simulink model "pruebas_of_modelo_completo"  (R2021a)
settings: Solver=VariableStepAuto  StartTime=0.0  StopTime=10.0  RelTol=1e-3
undefined symbols (not defined in the file): bah, bat, bcx, bcy, beqh, beqhd, beqt, bw, cont_mass, ddxmax, ddxmin, g, Kcy, Ksah, Ksat, Ksiah, Ksiat, Kw, Meqh, Meqt, Rd, rt, rth, Rw, sp_mass, yt0
settings Model: Creator=Mariano  LastModifiedBy=facu_

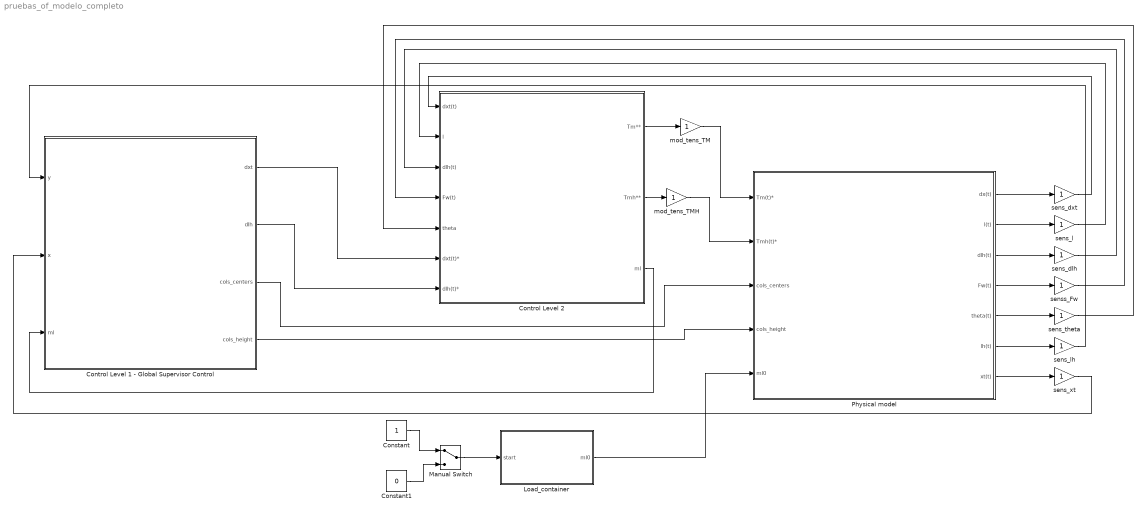
== system pruebas_of_modelo_completo ==
  Constant : Constant
  Constant1 : Constant  Value=0
  Control Level 1 - Global Supervisor Control : Stateflow chart  TreatAsAtomicUnit=on
  Control Level 2 : Subsystem
  Load_container : Subsystem
  Manual Switch : ManualSwitch
  Physical model : Subsystem
  mod_tens_TM : Gain
  mod_tens_TMH : Gain
  sens_dlh : Gain
  sens_dxt : Gain
  sens_l : Gain
  sens_lh : Gain
  sens_theta : Gain
  sens_xt : Gain
  senss_Fw : Gain
  wires:
  Control Level 2/1(Tm**) -> mod_tens_TM/1
  Control Level 2/2(Tmh**) -> mod_tens_TMH/1
  Control Level 1 - Global Supervisor Control/1(dxt) -> Control Level 2/6(dxt(t)*)
  Control Level 1 - Global Supervisor Control/2(dlh) -> Control Level 2/7(dlh(t)*)
  Physical model/1(dx(t)) -> sens_dxt/1
  Physical model/2(l(t)) -> sens_l/1
  Physical model/3(dlh(t)) -> sens_dlh/1
  Physical model/4(Fw(t)) -> senss_Fw/1
  Physical model/5(theta(t)) -> sens_theta/1
  Physical model/6(lh(t)) -> sens_lh/1
  Physical model/7(xt(t)) -> sens_xt/1
  sens_dxt/1 -> Control Level 2/1(dxt(t))
  sens_l/1 -> Control Level 2/2(l)
  sens_dlh/1 -> Control Level 2/3(dlh(t))
  senss_Fw/1 -> Control Level 2/4(Fw(t))
  sens_theta/1 -> Control Level 2/5(theta)
  sens_lh/1 -> Control Level 1 - Global Supervisor Control/1(y)
  sens_xt/1 -> Control Level 1 - Global Supervisor Control/2(x)
  mod_tens_TM/1 -> Physical model/1(Tm(t)*)
  mod_tens_TMH/1 -> Physical model/2(Tmh(t)*)
  Control Level 1 - Global Supervisor Control/3(cols_centers) -> Physical model/3(cols_centers)
  Control Level 1 - Global Supervisor Control/4(cols_height) -> Physical model/4(cols_height)
  Load_container/1(ml0) -> Physical model/5(ml0)
  Manual Switch/1 -> Load_container/1(start)
  Constant/1 -> Manual Switch/1
  Constant1/1 -> Manual Switch/2
  Control Level 2/3(ml) -> Control Level 1 - Global Supervisor Control/3(ml)

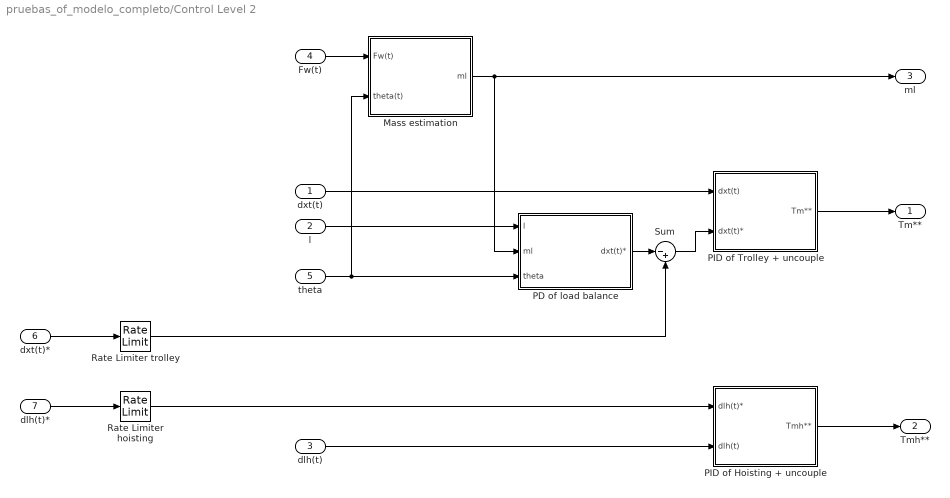
== system pruebas_of_modelo_completo/Control Level 2 ==
  dxt(t) : Inport
  l : Inport  Port=2
  dlh(t) : Inport  Port=3
  Fw(t) : Inport  Port=4
  theta : Inport  Port=5
  dxt(t)* : Inport  Port=6
  dlh(t)* : Inport  Port=7
  Mass estimation : Subsystem
  "PD of load balance " : Subsystem
  "PID of Hoisting + uncouple " : Subsystem
  "PID of Trolley + uncouple " : Subsystem
  Rate Limiter hoisting : RateLimiter  RisingSlewLimit=ddxmax  FallingSlewLimit=ddxmin
  Rate Limiter trolley : RateLimiter  RisingSlewLimit=ddxmax  FallingSlewLimit=ddxmin
  Sum : Sum  Inputs=|-+
  Tm** : Outport
  Tmh** : Outport  Port=2
  ml : Outport  Port=3
  wires:
  dlh(t)*/1 -> Rate Limiter hoisting/1
  Fw(t)/1 -> Mass estimation/1(Fw(t))
  "PID of Trolley + uncouple "/1(Tm**) -> Tm**/1
  Mass estimation/1(ml) -> ml/1, "PD of load balance "/2(ml)
  "PD of load balance "/1(dxt(t)*) -> Sum/1
  Sum/1 -> "PID of Trolley + uncouple "/2(dxt(t)*)
  dxt(t)/1 -> "PID of Trolley + uncouple "/1(dxt(t))
  "PID of Hoisting + uncouple "/1(Tmh**) -> Tmh**/1
  dxt(t)*/1 -> Rate Limiter trolley/1
  l/1 -> "PD of load balance "/1(l)
  theta/1 -> Mass estimation/2(theta(t)), "PD of load balance "/3(theta)
  Rate Limiter trolley/1 -> Sum/2
  Rate Limiter hoisting/1 -> "PID of Hoisting + uncouple "/1(dlh(t)*)
  dlh(t)/1 -> "PID of Hoisting + uncouple "/2(dlh(t))

== system pruebas_of_modelo_completo/Load_container ==
  start : Inport
  Sum : Sum  Inputs=|++
  Switch : Switch  Criteria=u2 > Threshold
  no_container : Constant  Value=0
  random_container_mass : Constant  Value=cont_mass
  spreader mass : Constant  Value=sp_mass
  ml0 : Outport
  wires:
  no_container/1 -> Switch/1
  spreader mass/1 -> Sum/2
  random_container_mass/1 -> Switch/3
  Switch/1 -> Sum/1
  Sum/1 -> ml0/1
  start/1 -> Switch/2

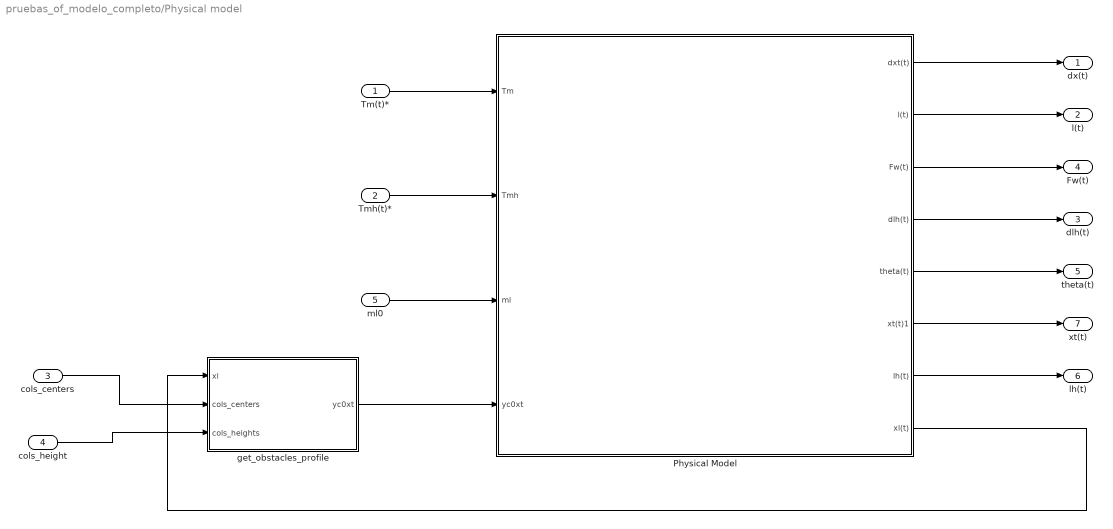
== system pruebas_of_modelo_completo/Physical model ==
  Tm(t)* : Inport
  Tmh(t)* : Inport  Port=2
  cols_centers : Inport  Port=3
  cols_height : Inport  Port=4
  ml0 : Inport  Port=5
  Physical Model : Subsystem
  get_obstacles_profile : MATLAB Function  TreatAsAtomicUnit=on
  dx(t) : Outport
  l(t) : Outport  Port=2
  dlh(t) : Outport  Port=3
  Fw(t) : Outport  Port=4
  theta(t) : Outport  Port=5
  lh(t) : Outport  Port=6
  xt(t) : Outport  Port=7
  wires:
  Physical Model/4(dlh(t)) -> dlh(t)/1
  Physical Model/2(l(t)) -> l(t)/1
  Physical Model/1(dxt(t)) -> dx(t)/1
  Physical Model/3(Fw(t)) -> Fw(t)/1
  Physical Model/5(theta(t)) -> theta(t)/1
  Physical Model/6(xt(t)1) -> xt(t)/1
  Physical Model/7(lh(t)) -> lh(t)/1
  Tmh(t)*/1 -> Physical Model/2(Tmh)
  Tm(t)*/1 -> Physical Model/1(Tm)
  ml0/1 -> Physical Model/3(ml)
  get_obstacles_profile/1(yc0xt) -> Physical Model/4(yc0xt)
  Physical Model/8(xl(t)) -> get_obstacles_profile/1(xl)
  cols_centers/1 -> get_obstacles_profile/2(cols_centers)
  cols_height/1 -> get_obstacles_profile/3(cols_heights)

== system pruebas_of_modelo_completo/Control Level 2/Mass estimation ==
  Fw(t) : Inport
  theta(t) : Inport  Port=2
  Constant : Constant  Value=g
  Divide : Product  Inputs=*/
  Product : Product
  Trigonometric Function : Trigonometry
  ml : Outport
  wires:
  theta(t)/1 -> Trigonometric Function/1
  Trigonometric Function/1 -> Product/2
  Fw(t)/1 -> Product/1
  Divide/1 -> ml/1
  Product/1 -> Divide/1
  Constant/1 -> Divide/2

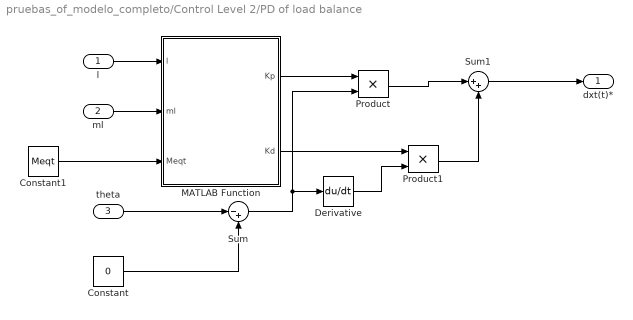
== system pruebas_of_modelo_completo/Control Level 2/PD of load balance  ==
  l : Inport
  ml : Inport  Port=2
  theta : Inport  Port=3
  Constant : Constant  Value=0
  Constant1 : Constant  Value=Meqt
  Derivative : Derivative
  MATLAB Function : MATLAB Function  TreatAsAtomicUnit=on
  Product : Product
  Product1 : Product
  Sum : Sum  Inputs=|-+
  Sum1 : Sum  Inputs=|++
  dxt(t)* : Outport
  wires:
  theta/1 -> Sum/1
  Constant/1 -> Sum/2
  ml/1 -> MATLAB Function/2(ml)
  Sum/1 -> Product/2, Derivative/1
  Product1/1 -> Sum1/2
  Product/1 -> Sum1/1
  Sum1/1 -> dxt(t)*/1
  MATLAB Function/2(Kd) -> Product1/1
  MATLAB Function/1(Kp) -> Product/1
  Derivative/1 -> Product1/2
  l/1 -> MATLAB Function/1(l)
  Constant1/1 -> MATLAB Function/3(Meqt)

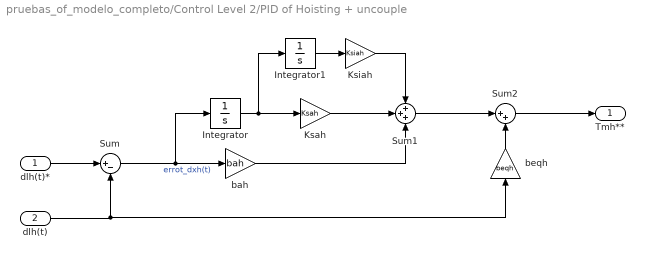
== system pruebas_of_modelo_completo/Control Level 2/PID of Hoisting + uncouple  ==
  dlh(t)* : Inport
  dlh(t) : Inport  Port=2
  Integrator : Integrator
  Integrator1 : Integrator
  Ksah : Gain  Gain=Ksah
  Ksiah : Gain  Gain=Ksiah
  Sum : Sum  Inputs=|+-
  Sum1 : Sum  Inputs=+++
  Sum2 : Sum  Inputs=|++
  bah : Gain  Gain=bah
  beqh : Gain  Gain=beqh
  Tmh** : Outport
  wires:
  Sum/1 -> bah/1, Integrator/1  "errot_dxh(t)"
  dlh(t)*/1 -> Sum/1
  Sum1/1 -> Sum2/1
  dlh(t)/1 -> beqh/1, Sum/2
  Integrator/1 -> Integrator1/1, Ksah/1
  bah/1 -> Sum1/3
  Ksah/1 -> Sum1/2
  Integrator1/1 -> Ksiah/1
  Ksiah/1 -> Sum1/1
  beqh/1 -> Sum2/2
  Sum2/1 -> Tmh**/1

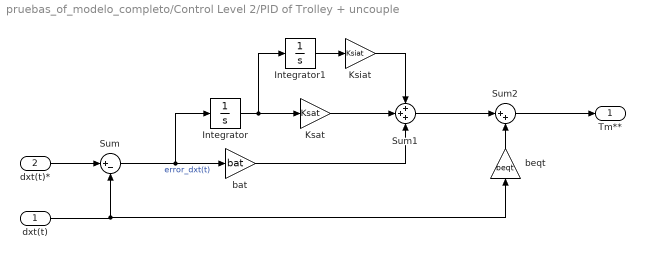
== system pruebas_of_modelo_completo/Control Level 2/PID of Trolley + uncouple  ==
  dxt(t) : Inport
  dxt(t)* : Inport  Port=2
  Integrator : Integrator
  Integrator1 : Integrator
  Ksat : Gain  Gain=Ksat
  Ksiat : Gain  Gain=Ksiat
  Sum : Sum  Inputs=|+-
  Sum1 : Sum  Inputs=+++
  Sum2 : Sum  Inputs=|++
  bat : Gain  Gain=bat
  beqt : Gain  Gain=beqt
  Tm** : Outport
  wires:
  Sum/1 -> bat/1, Integrator/1  "error_dxt(t)"
  dxt(t)*/1 -> Sum/1
  Sum1/1 -> Sum2/1
  dxt(t)/1 -> beqt/1, Sum/2
  Integrator/1 -> Integrator1/1, Ksat/1
  bat/1 -> Sum1/3
  Ksat/1 -> Sum1/2
  Integrator1/1 -> Ksiat/1
  Ksiat/1 -> Sum1/1
  beqt/1 -> Sum2/2
  Sum2/1 -> Tm**/1

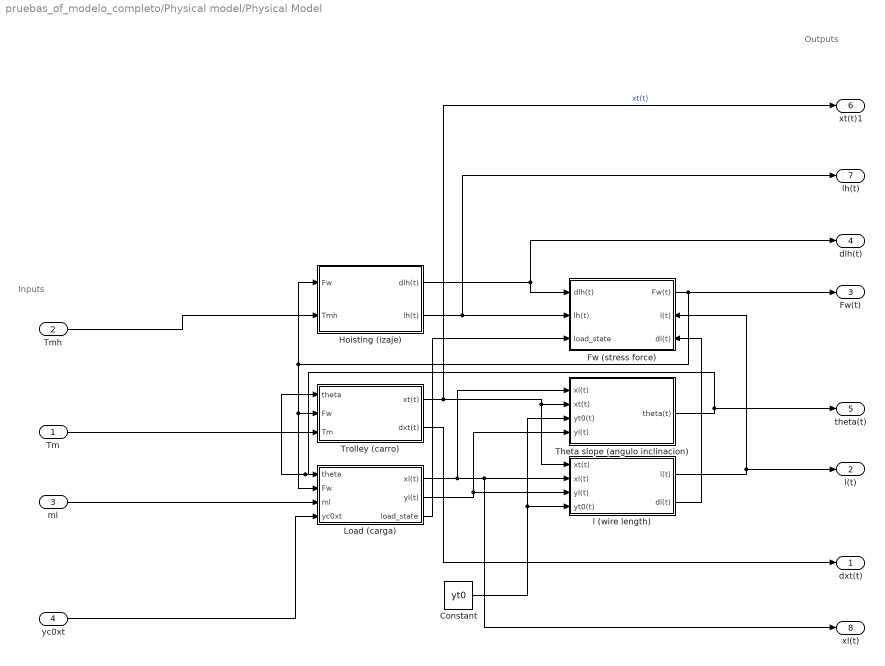
== system pruebas_of_modelo_completo/Physical model/Physical Model ==
  note: Inputs
  note: Outputs
  Tm : Inport
  Tmh : Inport  Port=2
  ml : Inport  Port=3
  yc0xt : Inport  Port=4
  Constant : Constant  Value=yt0
  Fw (stress force) : Subsystem
      settings: PortSchema="{\"entries\":[{\"content\":{\"sides\":[{\"content\":{\"connectorIds\":[\"In1\",\"In2\",\"In3\"]},\"type\":\"ConnectorPlacement.EquallySpacedRectSide\",\"uuid\":\"ba23d8a5-df88-4a98-9228-1a95ef0572d6\"},{\"content\":{\"connectorIds\":[\"Out1\",\"In4\",\"In5\"],\"side\":\"RIGHT\"},\"type\":\"ConnectorPlacement.EquallySpacedRectSide\",\"uuid\":\"c1b2cc2a-1d19-40da-89ec-405abbf25b58\"},{\"content\":{\"connectorIds\":[],\"side\":\"TOP\"},\"type\":\"ConnectorPlacement.EquallySpacedRectSide\",\"uuid\":\"8c283652-7118-429a-8320-3bc0966db205\"}]},\"type\":\"ConnectorPlacement.EquallySpacedConnector\",\"uuid\":\"7ebc4a5f-6f80-4333-9ee6-9a21b2f2a5d0\"}],\"packageUris\":[\"http://schema.mathworks.com/mf0/Connector/R2020b\"],\"version\":\"1.0\"}"
  Hoisting (izaje) : Subsystem
  Load (carga) : Subsystem
  Theta slope (angulo inclinacion) : Subsystem
  Trolley (carro) : Subsystem
  l (wire length) : Subsystem
  dxt(t) : Outport
  l(t) : Outport  Port=2
  Fw(t) : Outport  Port=3
  dlh(t) : Outport  Port=4
  theta(t) : Outport  Port=5
  xt(t)1 : Outport  Port=6
  lh(t) : Outport  Port=7
  xl(t) : Outport  Port=8
  wires:
  Theta slope (angulo inclinacion)/1(theta(t)) -> theta(t)/1, Trolley (carro)/1(theta), Load (carga)/1(theta)
  Load (carga)/1(xl(t)) -> xl(t)/1, l (wire length)/2(xl(t)), Theta slope (angulo inclinacion)/1(xl(t))
  Hoisting (izaje)/2(lh(t)) -> lh(t)/1, Fw (stress force)/2(lh(t))
  Trolley (carro)/1(xt(t)) -> xt(t)1/1, l (wire length)/1(xt(t)), Theta slope (angulo inclinacion)/2(xt(t))  "xt(t)"
  Fw (stress force)/1(Fw(t)) -> Trolley (carro)/2(Fw), Load (carga)/2(Fw), Hoisting (izaje)/1(Fw), Fw(t)/1
  Constant/1 -> Theta slope (angulo inclinacion)/3(yt0(t)), l (wire length)/4(yt0(t))
  Load (carga)/2(yl(t)) -> Theta slope (angulo inclinacion)/4(yl(t)), l (wire length)/3(yl(t))
  l (wire length)/1(l(t)) -> l(t)/1, Fw (stress force)/4(l(t))
  ml/1 -> Load (carga)/3(ml)
  l (wire length)/2(dl(t)) -> Fw (stress force)/5(dl(t))
  Tmh/1 -> Hoisting (izaje)/2(Tmh)
  Tm/1 -> Trolley (carro)/3(Tm)
  Hoisting (izaje)/1(dlh(t)) -> Fw (stress force)/1(dlh(t)), dlh(t)/1
  Trolley (carro)/2(dxt(t)) -> dxt(t)/1
  Load (carga)/3(load_state) -> Fw (stress force)/3(load_state)
  yc0xt/1 -> Load (carga)/4(yc0xt)

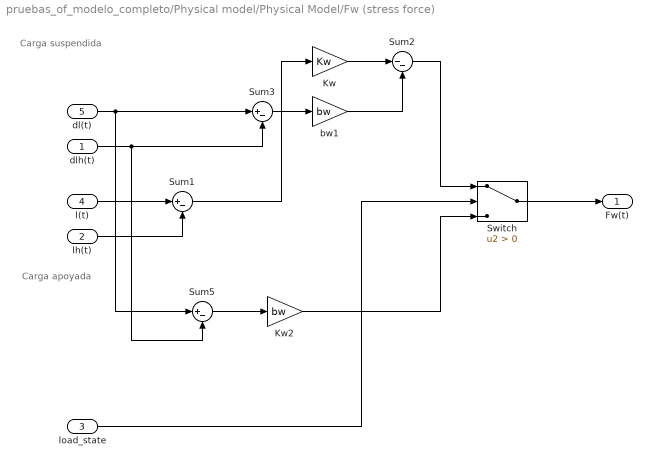
== system pruebas_of_modelo_completo/Physical model/Physical Model/Fw (stress force) ==
  note: Carga suspendida
  note: Carga apoyada
  dlh(t) : Inport
  lh(t) : Inport  Port=2
  load_state : Inport  Port=3
  l(t) : Inport  Port=4
  dl(t) : Inport  Port=5
  Kw : Gain  Gain=Kw
  Kw2 : Gain  Gain=bw
  Sum1 : Sum  Inputs=|+-
  Sum2 : Sum  Inputs=|--
  Sum3 : Sum  Inputs=|+-
  Sum5 : Sum  Inputs=|+-
  Switch : Switch  Criteria=u2 > Threshold
  bw1 : Gain  Gain=bw
  Fw(t) : Outport
  wires:
  Switch/1 -> Fw(t)/1
  l(t)/1 -> Sum1/1
  lh(t)/1 -> Sum1/2
  Sum1/1 -> Kw/1
  Sum3/1 -> bw1/1
  bw1/1 -> Sum2/2
  Kw/1 -> Sum2/1
  Sum2/1 -> Switch/1
  Sum5/1 -> Kw2/1
  dlh(t)/1 -> Sum5/2, Sum3/2
  dl(t)/1 -> Sum5/1, Sum3/1
  Kw2/1 -> Switch/3
  load_state/1 -> Switch/2

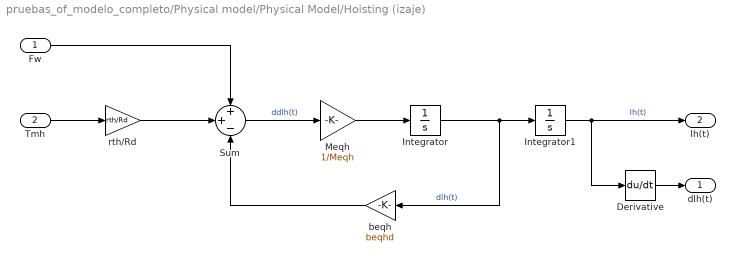
== system pruebas_of_modelo_completo/Physical model/Physical Model/Hoisting (izaje) ==
  Fw : Inport
  Tmh : Inport  Port=2
  Derivative : Derivative
  Integrator : Integrator
  Integrator1 : Integrator
  Meqh : Gain  Gain=1/Meqh
  Sum : Sum  Inputs=++-
  beqh : Gain  Gain=beqhd
  rth/Rd : Gain  Gain=rth/Rd
  dlh(t) : Outport
  lh(t) : Outport  Port=2
  wires:
  Fw/1 -> Sum/1
  Tmh/1 -> rth/Rd/1
  rth/Rd/1 -> Sum/2
  Sum/1 -> Meqh/1  "ddlh(t)"
  Meqh/1 -> Integrator/1
  Integrator/1 -> beqh/1, Integrator1/1  "dlh(t)"
  Integrator1/1 -> Derivative/1, lh(t)/1  "lh(t)"
  beqh/1 -> Sum/3
  Derivative/1 -> dlh(t)/1

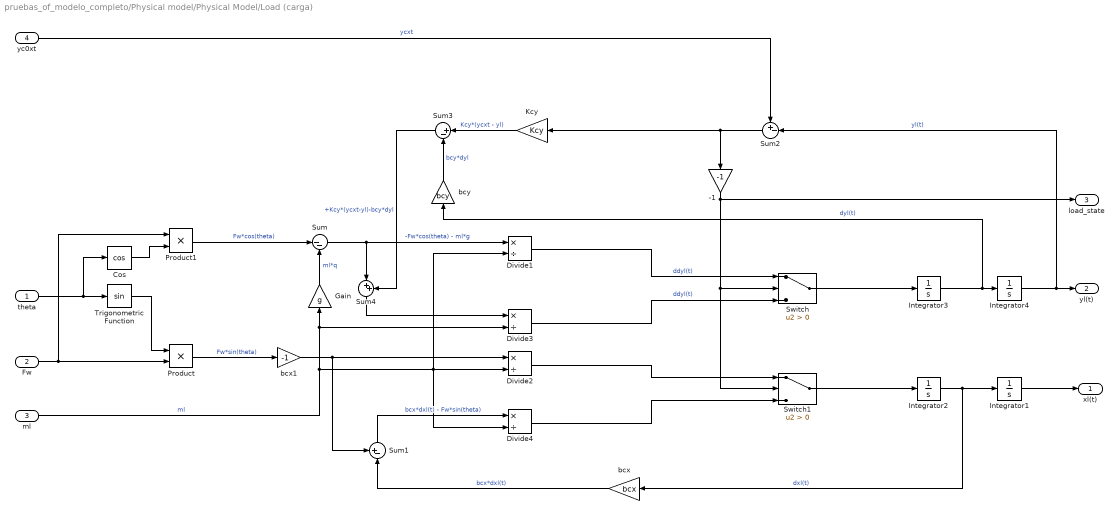
== system pruebas_of_modelo_completo/Physical model/Physical Model/Load (carga) ==
  theta : Inport
  Fw : Inport  Port=2
  ml : Inport  Port=3
  yc0xt : Inport  Port=4
  -1 : Gain  Gain=-1
  Cos : Trigonometry  Operator=cos
  Divide{1..4} (4 alike) : Product  Inputs=*/
  Gain : Gain  Gain=g
  Integrator{1..4} (4 alike) : Integrator
  Kcy : Gain  Gain=Kcy
  Product : Product
  Product1 : Product
  Sum : Sum  Inputs=|--
  Sum1 : Sum  Inputs=+-|
  Sum2 : Sum  Inputs=+-|
  Sum3 : Sum  Inputs=|+-
  Sum4 : Sum  Inputs=|++
  Switch : Switch  Criteria=u2 > Threshold
  Switch1 : Switch  Criteria=u2 > Threshold
  Trigonometric Function : Trigonometry
  bcx : Gain  Gain=bcx
  bcx1 : Gain  Gain=-1
  bcy : Gain  Gain=bcy
  xl(t) : Outport
  yl(t) : Outport  Port=2
  load_state : Outport  Port=3
  wires:
  theta/1 -> Trigonometric Function/1, Cos/1
  Trigonometric Function/1 -> Product/1
  Fw/1 -> Product/2, Product1/1
  Integrator1/1 -> xl(t)/1
  Integrator2/1 -> bcx/1, Integrator1/1  "dxl(t)"
  ml/1 -> Divide4/2, Divide2/2, Divide1/2, Divide3/2, Gain/1  "ml"
  Product/1 -> bcx1/1  "Fw*sin(theta)"
  Cos/1 -> Product1/2
  Product1/1 -> Sum/1  "Fw*cos(theta)"
  Sum/1 -> Sum4/1, Divide1/1  "-Fw*cos(theta) - ml*g"
  Integrator3/1 -> bcy/1, Integrator4/1  "dyl(t)"
  Integrator4/1 -> Sum2/2, yl(t)/1  "yl(t)"
  Gain/1 -> Sum/2  "ml*q"
  Divide1/1 -> Switch/1  "ddyl(t)"
  Switch/1 -> Integrator3/1
  Switch1/1 -> Integrator2/1
  Divide2/1 -> Switch1/1
  Divide4/1 -> Switch1/3
  Divide3/1 -> Switch/3  "ddyl(t)"
  bcx1/1 -> Sum1/1, Divide2/1
  bcx/1 -> Sum1/2  "bcx*dxl(t)"
  Sum1/1 -> Divide4/1  "bcx*dxl(t) - Fw*sin(theta)"
  Sum2/1 -> Kcy/1, -1/1
  yc0xt/1 -> Sum2/1  "ycxt"
  Kcy/1 -> Sum3/1  "Kcy*(ycxt - yl)"
  bcy/1 -> Sum3/2  "bcy*dyl"
  Sum4/1 -> Divide3/1
  Sum3/1 -> Sum4/2  "+Kcy*(ycxt-yl)-bcy*dyl"
  -1/1 -> load_state/1, Switch1/2, Switch/2

== system pruebas_of_modelo_completo/Physical model/Physical Model/Theta slope (angulo inclinacion) ==
  xl(t) : Inport
  xt(t) : Inport  Port=2
  yt0(t) : Inport  Port=3
  yl(t) : Inport  Port=4
  Atan2 : Trigonometry  Operator=atan2
  Sum : Sum  Inputs=-+
  Sum1 : Sum  Inputs=+-
  theta(t) : Outport
  wires:
  yt0(t)/1 -> Sum/1
  yl(t)/1 -> Sum/2
  xl(t)/1 -> Sum1/1
  xt(t)/1 -> Sum1/2
  Sum1/1 -> Atan2/1  "xl-xt"
  Sum/1 -> Atan2/2  "yl-yt"
  Atan2/1 -> theta(t)/1

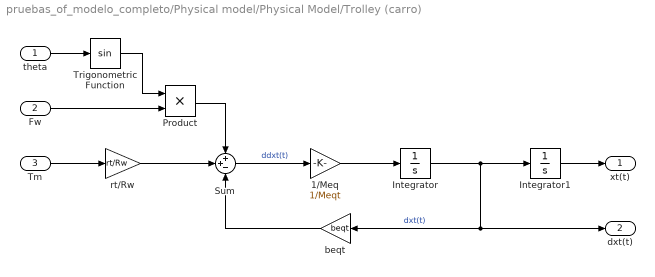
== system pruebas_of_modelo_completo/Physical model/Physical Model/Trolley (carro) ==
  theta : Inport
  Fw : Inport  Port=2
  Tm : Inport  Port=3
  1/Meq : Gain  Gain=1/Meqt
  Integrator : Integrator
  Integrator1 : Integrator
  Product : Product
  Sum : Sum  Inputs=++-
  Trigonometric Function : Trigonometry
  beqt : Gain  Gain=beqt
  rt/Rw : Gain  Gain=rt/Rw
  xt(t) : Outport
  dxt(t) : Outport  Port=2
  wires:
  theta/1 -> Trigonometric Function/1
  Trigonometric Function/1 -> Product/1
  Fw/1 -> Product/2
  Product/1 -> Sum/1
  Tm/1 -> rt/Rw/1
  rt/Rw/1 -> Sum/2
  Sum/1 -> 1/Meq/1  "ddxt(t)"
  1/Meq/1 -> Integrator/1
  Integrator/1 -> Integrator1/1, dxt(t)/1, beqt/1  "dxt(t)"
  Integrator1/1 -> xt(t)/1
  beqt/1 -> Sum/3

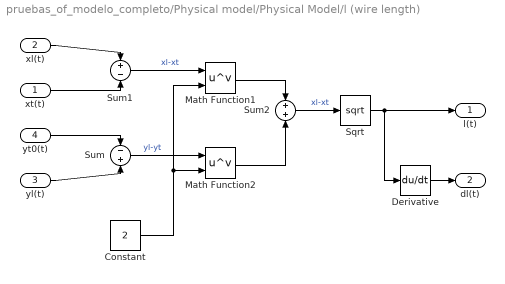
== system pruebas_of_modelo_completo/Physical model/Physical Model/l (wire length) ==
  xt(t) : Inport
  xl(t) : Inport  Port=2
  yl(t) : Inport  Port=3
  yt0(t) : Inport  Port=4
  Constant : Constant  Value=2
  Derivative : Derivative
  Math Function1 : Math  Operator=pow  SignedPower=on  SaturateOnIntegerOverflow=on
  Math Function2 : Math  Operator=pow  SignedPower=on  SaturateOnIntegerOverflow=on
  Sqrt : Sqrt  SaturateOnIntegerOverflow=on
  Sum : Sum  Inputs=-+
  Sum1 : Sum  Inputs=+-
  Sum2 : Sum
  l(t) : Outport
  dl(t) : Outport  Port=2
  wires:
  yt0(t)/1 -> Sum/1
  yl(t)/1 -> Sum/2
  xl(t)/1 -> Sum1/1
  xt(t)/1 -> Sum1/2
  Sqrt/1 -> Derivative/1, l(t)/1
  Sum1/1 -> Math Function1/1  "xl-xt"
  Sum/1 -> Math Function2/1  "yl-yt"
  Math Function1/1 -> Sum2/1
  Math Function2/1 -> Sum2/2
  Sum2/1 -> Sqrt/1  "xl-xt"
  Derivative/1 -> dl(t)/1
  Constant/1 -> Math Function2/2, Math Function1/2

== matlab function pruebas_of_modelo_completo/Control Level 2/PD of load balance /MATLAB Function ==
  data: l input; Kp output; ml input; Kd output; Meqt input
function [Kp,Kd] = fcn(l, ml,Meqt)
    wn=800;
    g=9.81;
    Kd = l - ( (Meqt*g)/((wn^2)*(ml+Meqt)) ) ;
    Kp = 2*wn*1*(-l + Kd);
end

== stateflow chart pruebas_of_modelo_completo/Control Level 1 - Global Supervisor Control ==
  note: Descripcion variables:
      | CARRO (TROLLEY):
      | - move_t -> (variable,int) boton para mover el carro en x.
      | - dx -> (variable,double) velocidad actual del carro (variable)
      | - VXt -> velocidad máxima del carro (es una constante, que al multiplicarla por bot_t modifica el valor de la velocidad real de carro.)
      | - limits_t -> (variable,bool) la variable cambia al valor 1 si se alcanzan los limites de movimiento del carro.
      |
      | IZAJE (HOISTING):
      | - move_h ->(variable,int) boton para izar la carga.
      | - dy -> (variable,double) velocidad actual del izaje.
      | - VYh -> (constante) velocidad máxima que puede alcanzar el izaje.
      | - limits_h -> (variable,bool) la variable cambia al valor 1 si se alcanzan los limites de movimiento del izaje.
      |
      | Descripcion de bloques:
      | - ALL_MANUAL:
      | Es el modo manual por defecto, el operario puede manejar el trolley y el hoisting con 2 botones. El boton move_t se encarga de mover el trolley y el boton move_h de izar la carga.
      | - HYRBID_MANUAL:
      | Es el modo manual que esta presente en los ciclos simple o doble. Es decir, esta intercalado con el modo automático
  note: Descripción de ciclos:
      | -SIMPLE:
      | O se carga o se descarga, es decir: Si estoy cargando el barco, en el tramo muelle -> barco llevo un contenedor, pero vuelvo vacio. Es decir que el tramo barco -> muelle es sin ningun contenedor. Lo mismo sucederia si estoy descargando el barco: el tramo barco -> muelle es con un contenedor cargado, pero el tramo muelle -> barco es en vacio.
      | - DOBLE:
      | Se puede cargar y descargar en el mismo ciclo de trabajo. Es decir, que el tramo muelle -> barco es con un contenedor cargado, y el tramo barco -> muelle también. Por ende, se permite una carga intermedia antes de volver al muelle.
      |
      | ETAPAS DE LA TRAYECTORIA:
      | Cada stage se va aactivando dependiendo del punto de la trayectoria en el que se encuentra el barco
      | - STAGE 1 -> ground - el contenedor esta en tierra
      | - STAGE 2 -> el contenedor se encuentra en el aire (sobre muelle), en el punto de transicion manual a automatico.
      | - STAGE 3 -> el contenedor se enceuntra en el aire (sobre barco) ,en el punto de transicion automatico a manual.
      | - STAGE 4 -> el contenedor se encuentra en el barco.
  state LEVEL1
    entry: [p00,p11,p22,p33,p44,p55,p66,p77,cols_h,cols_c,VH,VT,double,single] = generate_trajectory(23562,"to_ship","single");
    auto_mode=1,p0=p00,p1=p11,p2=p22,p3=p33,p4=p44,p5=p55,p6=p66,p7=p77;
    cols_height=cols_h,cols_centers=cols_c,VH_MAX=VH,VT_MAX=VT,cycle_double=double,cycle_single=single;
    during: getcharge=get_charge(ml),charge=getcharge;
    state MOVEMENT [parallel]
      settings: executionOrder=2
      state MANUAL
        entry: joy_t=0.9, joy_h=0.9, dxt=0,dlh=0;
        state HYBRID_MANUAL
          state HOISTING [parallel]
            entry: limits_h=0;
            settings: executionOrder=1
            state MOVE
              during:
              dlh=1;
            state STOP
              entry:
              dlh=0;
            (default) -> LEVEL1.MOVEMENT.MANUAL.HYBRID_MANUAL.HOISTING.MOVE
            LEVEL1.MOVEMENT.MANUAL.HYBRID_MANUAL.HOISTING.STOP -> LEVEL1.MOVEMENT.MANUAL.HYBRID_MANUAL.HOISTING.MOVE : [joy_h~=0 || limits_h==0]
            LEVEL1.MOVEMENT.MANUAL.HYBRID_MANUAL.HOISTING.MOVE -> LEVEL1.MOVEMENT.MANUAL.HYBRID_MANUAL.HOISTING.STOP : [joy_h==0 || limits_h==1]
          state TROLLEY [parallel]
            entry: limits_t=0;
            settings: executionOrder=2
            state STOP
              entry:
              dxt=0;
            state MOVE
              during:
              dxt=1;
            (default) -> LEVEL1.MOVEMENT.MANUAL.HYBRID_MANUAL.TROLLEY.MOVE
            LEVEL1.MOVEMENT.MANUAL.HYBRID_MANUAL.TROLLEY.STOP -> LEVEL1.MOVEMENT.MANUAL.HYBRID_MANUAL.TROLLEY.MOVE : [joy_t~=0 || limits_t==0]
            LEVEL1.MOVEMENT.MANUAL.HYBRID_MANUAL.TROLLEY.MOVE -> LEVEL1.MOVEMENT.MANUAL.HYBRID_MANUAL.TROLLEY.STOP : [joy_t==0 || limits_t==1]
        (default) -> HYBRID_MANUAL
      state AUTOMATIC
        entry: bot_cy=0;
        state TO_SHIP
          during:
          dxt = VT_MAX*0.6;
          dlh = VH_MAX*0.6;
          if single_cycle && charge == 0
          dxt = VH_MAX;
          dlh = VT_MAX;
          end
        state INIT
        state TO_DOCK
          during:
          dxt = VT_MAX*0.6;
          dlh = VH_MAX*0.6;
          if single_cycle && charge == 1
          dxt = VT_MAX;
          dlh = VH_MAX;
          end
        LEVEL1.MOVEMENT.AUTOMATIC.INIT -> TO_SHIP [order 1] : [current_stage == 1 && prev_stage == 0]
        (default) -> LEVEL1.MOVEMENT.AUTOMATIC.INIT
        LEVEL1.MOVEMENT.AUTOMATIC.INIT -> TO_DOCK [order 2] : [current_stage == 6 && prev_stage == 7]
      (default) -> MANUAL
      HYBRID_MANUAL -> AUTOMATIC [order 1] : [(current_stage ==  1 && prev_stage == 0) && auto_mode == 1 && ( single_cycle==1 || (double_cycle==1 && charge==1))]
      HYBRID_MANUAL -> AUTOMATIC [order 2] : [current_stage == 6 && prev_stage == 7 && auto_mode == 1 && ( single_cycle==1 || (double_cycle==1 && charge==1)) ]
      TO_SHIP -> HYBRID_MANUAL : [current_stage == 6 && prev_stage == 5]
      AUTOMATIC -> MANUAL : [joy_t~=0 || joy_h~=0]
      TO_DOCK -> HYBRID_MANUAL : [current_stage == 1 && prev_stage == 2]
    state TRAJECTORY [parallel]
      settings: executionOrder=1
      state STAGE_7
        during:
        current_stage=7;
        exit:
        prev_stage=7;
      state INIT
      state STAGE_0
        during:
        current_stage = 0;
        exit:
        prev_stage=0;
      state STAGE_6
        during:
        current_stage=6;
        exit:
        prev_stage=6;
      state STAGE_1
        during:
        current_stage = 1;
        exit:
        prev_stage=1;
      state STAGE_5
        during:
        current_stage=5;
        exit:
        prev_stage=5;
      state STAGE_2
        during:
        current_stage = 2;
        exit:
        prev_stage=2;
      state STAGE_4
        during:
        current_stage=4;
        exit:
        prev_stage=4;
      state STAGE_3
        during:
        current_stage=3;
        exit:
        prev_stage=3;
      (default) -> LEVEL1.TRAJECTORY.INIT
      LEVEL1.TRAJECTORY.INIT -> STAGE_7 [order 2] : [y>=p7(2)&&x>=p7(1)]
      LEVEL1.TRAJECTORY.INIT -> STAGE_0 [order 1] : [(y>=p0(2) && x>=p0(1))]
      STAGE_0 -> STAGE_1 : [(y>=p1(2) && x>=p1(1))]
      STAGE_1 -> STAGE_0 [order 2] : [(y<=p0(2) && x<=p0(1))]
      STAGE_7 -> STAGE_6 : [y>=p6(2)&&x==p7(1)]
      STAGE_6 -> STAGE_7 [order 2] : [(y<=p7(2)&&x==p7(1))]
      STAGE_6 -> STAGE_5 [order 1] : [(y>=p5(2)&&x>=p5(1))]
      STAGE_5 -> STAGE_6 [order 2] : [(y<=p6(2)&&x>=p6(1))]
      STAGE_1 -> STAGE_2 [order 1] : [(y>=p2(2) && x>=p2(1))]
      STAGE_2 -> STAGE_1 [order 2] : [(y<=p1(2)&&x<=p1(1))]
      STAGE_2 -> STAGE_3 [order 1] : [(y>=p3(2)&&x>=p3(1))]
      STAGE_3 -> STAGE_2 [order 1] : [(y<=p2(2)&&x<=p2(1))]
      STAGE_5 -> STAGE_4 [order 1] : [(y>=p4(2)&&x<=p4(1))]
      STAGE_4 -> STAGE_5 [order 1] : [(y<=p5(2)&&x<=p5(1))]
      STAGE_4 -> STAGE_3 [order 2] : [(y<=p3(2)&&x<=p3(1))]
      STAGE_3 -> STAGE_4 [order 2] : [ (y>=p4(2)&&x>=p4(1))]
  (default) -> LEVEL1
  data: ml1 function_input; charge_ function_output; weight function_input; to_where function_input; cycle_type function_input; p0 function_output; p1 function_output; p2 function_output; p3 function_output; p4 function_output; p5 function_output; p6 function_output; p7 function_output; cols_height function_output; cols_centers function_output; VH_MAX function_output; VT_MAX function_output; double_cycle function_output; single_cycle function_output; dxt output size=2; dlh output size=2; y input; x input; cols_centers output; cols_height output; ml input; bot_cy local; VH_MAX local; VT_MAX local; auto_mode local; charge local; current_stage local; double_cycle local; joy_h local; joy_t local; limits_h local; limits_t local; p0 local; p1 local; p2 local; p3 local; p4 local; p5 local; p6 local; p7 local; prev_stage local; single_cycle local; getcharge local
  function charge_=get_charge(ml1):
    | function charge_=get_charge(ml1)
    | if ml1>1500
    |     charge_=1;
    | else
    |     charge_=0;
    | end
  function [p0,p1,p2,p3,p4,p5,p6,p7,cols_height,cols_centers,VH_MAX,VT_MAX,double_cycle,single_cycle] = generate_trajectory(weight,to_where,cycle_type):
    | function [p0,p1,p2,p3,p4,p5,p6,p7,cols_height,cols_centers,VH_MAX,VT_MAX,double_cycle,single_cycle] = generate_trajectory(weight,to_where,cycle_type)
    | 
    | init = 1;
    | plt_traj = "true";
    | if cycle_type=="single"
    |     double_cycle=0;
    |     single_cycle=1;
    | else
    |     double_cycle=1;
    |     single_cycle=0;
    | end
    | 
    | %% Defincion de los parametros iniciales previo a comenzar el trayecto
    | 
    | if init
    |     % Velocidades maximas a alcanzar por carro e izaje
    |     VT_MAX=4; %[m/s]
    |     VH_MAX=1.5; %[m/s]
    |     YSB=15;
    | 
    |     % Definimos dimensiones de un contendor maritimo [metros]
    |     C_HEIGHT = 2.89;
    |     C_WIDTH = 2.438;
    |     c_weight = weight;
    | 
    |     % Definimos dimensiones del barco (ship) [metros]
    |     S_WIDTH = 45;
    |     N_COLS = round(S_WIDTH/C_WIDTH); % Cantidad de columnas del barco
    |     MAX_C_OVER_DOCK= 9; % Cantidad maxima de containers sobre nivel del muelle
    |     MAX_C_UNDER_DOCK = 4; % cantidad de containers por debajo del nivel del muelle [metros]
    |     
    |     % Generamos de forma aleatoria columnas con diferentes alturas.
    |     cols_height = generate_cols_height(MAX_C_OVER_DOCK,N_COLS,C_HEIGHT,MAX_C_UNDER_DOCK);
    |     
    |     %Generamos array que contiene los centros de cada columna respecto al
    |     %muelle (punto 0,0)
    |     delta = 0; 
    |     cols_centers = find_cols_centers(C_WIDTH/2,delta,N_COLS);
    |     
    | end
    | 
    | %% Comienzo de generacion de la trayectoria dependiendo de la situacion
    | slope=atan(VH_MAX/VT_MAX); %pendiente
    | 
    | % Definimos el punto de inicio (p1) en el muelle con coordenadas x,y
    | p0=[-20,0];
    | 
    | % Generamos un numero aleatorio que nos dice a que numero de columna debemos llevar el contenedor. Definimos asi p6.
    | while(1)
    |     index_goal=randi([1,N_COLS],1,1);
    |     if cols_height(index_goal)<C_HEIGHT*MAX_C_OVER_DOCK
    |         break;
    |     end
    | end
    | %index_goal=1;
    | p7=[cols_centers(index_goal),cols_height(index_goal)];
    | 
    | % Generamos un vector que solo contenga las columnas a la izquierda del punto objetivo. Son los unicos puntos que importan.
    | left_cols=cols_height(1:index_goal);
    | 
    | % Buscamos los de las columnas de mayor altura , tanto la que se encuentra mas a la izquierda como la que se encuentra mas a la
    | % derecha.
    | max=0;
    | for i=1:index_goal
    |     if left_cols(i)>=max
    |         imax_right=i;
    |         if left_cols(i)>max
    |             imax_left=i;
    |         end
    |     max=left_cols(i);
    |     end
    | end
    | 
    | %% Calculo de p3 y p2
    | 
    | % Definimos la altura de seguridad que me definira la coord y de p3.
    | % Se considera la altura de 2 contenedores para seguridad
    | H_SAFE=max+2*C_HEIGHT;
    | 
    | % Definimos el x de seguridad, que define la coord. x de p3
    | % Se considera el ancho de un contenedor para seguridad
    | x_safe=cols_centers(imax_left)-C_WIDTH;
    | 
    | % Primer valor de p3, sin verificacion aun.
    | p3=[x_safe,H_SAFE];
    | 
    | % Definimos p2 usando trigonometria.
    | p2=[-20, p3(2)-tan(slope)*(p3(1)-p0(1))];
    | 
    | % Bucle que verifica que la trayectoria de p3 a p2 no con otra columna. Si esto ocurre, modificamos el valor de p3
    | % y por ende de p2.
    | e=0;
    | next_index=imax_left-1;
    | while next_index>0
    | 
    |    % y23 indica el valor de la recta que une p2 con p3 en el punto
    |    % central de cada columna.
    |    y23=p3(2)-tan(slope)*(p3(1)-cols_centers(next_index));
    | 
    |    % Verificamos que no haya colision entre la recta que une p2
    |    % con p3 (mas una distancia de seguridad) y la columna.
    |    if y23<cols_height(next_index)+2*C_HEIGHT
    | 
    |         % Si hay colision, entonces debemos actualizar p3 y por
    |         % ende, p2. Para actualizar p3 se corre un ancho a la
    |         % izquierda el punto x de p3.
    |         e=e+1;
    |         p3=[x_safe-e*C_WIDTH,H_SAFE];
    |         p2=[-20, p3(2)-tan(slope)*(p3(1)-p0(1))];
    |         next_index=imax_left;
    |    end
    |    next_index=next_index-1;
    | end
    | 
    | 
    | %%  Calculo de p4 y p5
    | 
    | % Si el contenedor tiene que ir a la primer columna, o tiene que ir
    | % a un maximo el p4 y p5 en x seran igual al p6 x. En altura seran
    | %la altura de seguridad
    | if (index_goal ==1 || max==left_cols(index_goal))
    |     p4=[p7(1),H_SAFE];
    |     p5=p4;
    | 
    | else
    |     % Definimos el x de seguridad, que define la coord. x de p3
    |     % Se considera el ancho de un contenedor para seguridad
    |     x_safe=cols_centers(imax_right)+C_WIDTH;
    | 
    |     % Primer valor de p4, sin verificacion aun.
    |     p4=[x_safe,H_SAFE];
    | 
    |     % Definimos p5 usando trigonometria.
    |     p5=[p7(1), p4(2)+tan(slope)*(p4(1)-p7(1))];
    |     % Bucle que verifica que la trayectoria de p4 a p5 no con otra
    |     % columna. Si esto ocurre, modificamos el valor de p4
    |     % y por ende de p5.
    |     e=0;
    |     next_index=imax_right+1;
    |     while next_index<=index_goal
    | 
    |        % y45 indica el valor de la recta que une p4 con p5 en el punto
    |        % central de cada columna.
    |        y45=p4(2)+tan(slope)*(p4(1)-cols_centers(next_index));
    | 
    |        % Verificamos que no haya colision entre la recta que une p4
    |        % con p5 (mas una distancia de seguridad) y la columna.
    |        if y45<cols_height(next_index)+2*C_HEIGHT
    | 
    |             % Si hay colision, entonces debemos actualizar p4 y por
    |             % ende, p5. Para actualizar p4 se corre un ancho a la
    |             % derecha el punto x de p4.
    |             e=e+1;
    |             p4=[x_safe+e*C_WIDTH,H_SAFE];
    |             p5=[p7(1), p4(2)+tan(slope)*(p4(1)-p7(1))];
    |             next_index=imax_right;
    |        end
    |        next_index=next_index+1;
    |     end
    | end
    | 
    | p1 = [p0(1),(p2(2)-p0(2))/2];
    | p6 = [p7(1),(p5(2)-p7(2))/2+p7(2)];
    | 
    | switch(to_where)    
    |     case 'to_ship' 
    |     % En este caso los puntos seran como se calcularon.
    |     
    |     case 'to_dock'       
    |     % En este caso se invierten los puntos, el p1 sera aleatorio y el p6
    |     % será un punto fijo en (-20,0). Primero guardamos los puntos en puntos
    |     % auxiliares y luego se actualizan.
    |     p0d=p0;
    |     p1d=p1;
    |     p2d=p2;
    |     p3d=p3;
    |     p4d=p4;
    |     p5d=p5;
    |     p6d=p6;
    |     p7d=p7;
    |     p7=p7d;
    |     p6=p1d;
    |     p5=p2d;
    |     p4=p3d;
    |     p3=p4d;
    |     p2=p5d;
    |     p1=p6d;
    |     p0=p0d;
    |    
    | end % end switch
    | 
    | %% Plot del perfil de trayectoria obtenido
    | hold on
    | if (plt_traj == "true")
    |     plot_containers(cols_height,cols_centers);
    |     plot(p0(1),p0(2),'ko')
    |     plot(p1(1),p1(2),'ko')
    |     plot([p2(1) p3(1)],[p2(2) p3(2)],'r')
    |     plot([p2(1) p3(1)],[p2(2) p3(2)],'ko')
    |     plot(p6(1),p6(2),'ko')
    |     plot(p7(1),p7(2),'bo')
    |     plot([p4(1) p5(1)],[p4(2) p5(2)],'r')
    |     plot([p4(1) p5(1)],[p4(2) p5(2)],'ko')
    | end %endif
    | 
    | points = [p0,p1,p2,p3,p4,p5,p6,p7];
    | yc0xt = cols_height;
    | 
    | end % end function
    | function [centers] = find_cols_centers(step,delta,n_cols)
    |     centers = [];
    |     for i=1:n_cols
    |         centers(1,i)= 2*step*i+delta-step;
    |     end
    | end
    | function [h_cols] = generate_cols_height(max_n_cnts,n_cols,c_height,c_under_dock)
    |     rng('shuffle')
    |     h_cols = c_height * randi([-c_under_dock,max_n_cnts],n_cols,1);
    | end
    | function [] = plot_containers(h_cols,centers)
    |     bar(centers,h_cols);
    | end

== matlab function pruebas_of_modelo_completo/Physical model/get_obstacles_profile ==
  data: xl input; yc0xt output; cols_centers input; cols_heights input
function yc0xt = get_obstacles_profile(xl, cols_centers, cols_heights)

%{
@type MATLAB function called from SIMULINK
@name get_obstacles_profile
@description - Obtiene el perfil de obstaculos 
@params {float,simulation} xl - valor en tiempo real de la posocion del
carro
@params {array} cols_centers - Contiene las coordenadas de los centros de
cada columna. Array de 1xN , con N = cantidad de columnas
@params {cols_heights} - Altura de cada columna respecto del punto 0,0.
@returns {float} yc0xt - Valor en altura del obstaculo para la coordenada
xl, en el instante de tiempo t actual.
%}


if (xl <= 0) % Si estamos sobre el muelle no hay obstaculos, entonces ycxt=0
    yc0xt = 0;

elseif (xl > 0) % Si estamos por encima del barco
    
    
end % end ifelse

end %end function
